simulink model "RegolazioneLQ_mdl"  (Simulink 8.1)
settings: Solver=ode45  StartTime=0.0  StopTime=10.0  RelTol=1e-3
values from neighbouring files (symbols this model uses):
  Dx0 = [0.05 0.01 0 0]'    [TSC150918ProvaMatlab.m]
undefined symbols (not defined in the file or in its folder): A, B, C, K
settings Model: Creator=lbiagiotti  LastModifiedBy=peppe
settings DebuggingCC: SolverPrmCheckMsg=none  StrictBusMsg=Warning

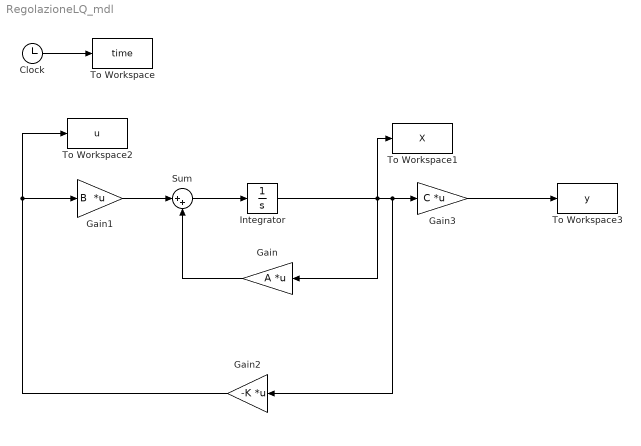
== system RegolazioneLQ_mdl ==
  Clock : Clock
  Gain : Gain  Gain=A  Multiplication=Matrix(K*u)
  Gain1 : Gain  Gain=B  Multiplication=Matrix(K*u)
  Gain2 : Gain  Gain=-K  Multiplication=Matrix(K*u)
  Gain3 : Gain  Gain=C  Multiplication=Matrix(K*u)
  Integrator : Integrator  InitialCondition=Dx0
  Sum : Sum  Inputs=|++
  To Workspace : ToWorkspace  VariableName=time  SampleTime=-1
  To Workspace1 : ToWorkspace  VariableName=X  SampleTime=-1
  To Workspace2 : ToWorkspace  VariableName=u  SampleTime=-1
  To Workspace3 : ToWorkspace  VariableName=y  SampleTime=-1
  wires:
  Integrator/1 -> To Workspace1/1, Gain/1, Gain3/1, Gain2/1
  Sum/1 -> Integrator/1
  Clock/1 -> To Workspace/1
  Gain3/1 -> To Workspace3/1
  Gain1/1 -> Sum/1
  Gain/1 -> Sum/2
  Gain2/1 -> Gain1/1, To Workspace2/1
